simulink library "halin"  (R2021b)
settings: Solver=VariableStepAuto  StartTime=0.0  StopTime=10.0  RelTol=1e-3
undefined symbols (not defined in the file): KHAL_CAN1ABM1E2E_flg, KHAL_CAN1ESC1E2E_flg, KHAL_CAN1ESC5E2E_flg, KHAL_CAN1ESC7E2E_flg, KHAL_CAN1FCM2E2E_flg, KHAL_CAN1FCM3E2E_flg, KHAL_CAN1FCM4E2E_flg, KHAL_CAN3BMS1E2E_flg, KHAL_CAN3BMS6E2E_flg, KHAL_CAN3CCU1E2E_flg, KHAL_CAN3CCU2E2E_flg, KHAL_CAN3MCUF1E2E_flg, KHAL_CAN3MCUR1E2E_flg, KHAL_CAN3Shifter1E2E_flg, TRUE
libraries: simulink x420, FVT_lib x149, hcu_lib x49
(part 14 of 14)

== system halin/HAL_IN/CAN3/MCU_R2/RrCoolanttempReq ==
  Rr_CoolanttempReq : Inport
  UnitConverter : DataTypeConversion  OutDataTypeStr=uint16
  convert_in : FVT_lib/hal/convert_in  gain=1  offset=-40
  VHAL_RrCoolanttempReq_cnt : Outport
  wires:
  convert_in/1 -> VHAL_RrCoolanttempReq_cnt/1
  UnitConverter/1 -> convert_in/1
  Rr_CoolanttempReq/1 -> UnitConverter/1

== system halin/HAL_IN/CAN3/MCU_R2/RrEOPSpdSet ==
  Rr_EOP_SpdSet : Inport
  UnitConverter : DataTypeConversion  OutDataTypeStr=uint16
  VHAL_RrEOPSpdSet_rpm : Outport
  wires:
  UnitConverter/1 -> VHAL_RrEOPSpdSet_rpm/1
  Rr_EOP_SpdSet/1 -> UnitConverter/1

== system halin/HAL_IN/CAN3/MCU_R2/RrFailcode1 ==
  Rr_Failcode1 : Inport
  UnitConverter : DataTypeConversion  OutDataTypeStr=uint8
  VHAL_RrFailcode1_enum : Outport
  wires:
  UnitConverter/1 -> VHAL_RrFailcode1_enum/1
  Rr_Failcode1/1 -> UnitConverter/1

== system halin/HAL_IN/CAN3/MCU_R2/RrFailcode2 ==
  Rr_Failcode2 : Inport
  UnitConverter : DataTypeConversion  OutDataTypeStr=uint8
  VHAL_RrFailcode2_enum : Outport
  wires:
  UnitConverter/1 -> VHAL_RrFailcode2_enum/1
  Rr_Failcode2/1 -> UnitConverter/1

== system halin/HAL_IN/CAN3/MCU_R2/RrFailcodehistory1 ==
  Rr_Failcodehistory1 : Inport
  UnitConverter : DataTypeConversion  OutDataTypeStr=uint8
  VHAL_RrFailcodehistory1_enum : Outport
  wires:
  UnitConverter/1 -> VHAL_RrFailcodehistory1_enum/1
  Rr_Failcodehistory1/1 -> UnitConverter/1

== system halin/HAL_IN/CAN3/MCU_R2/RrFailcodehistory2 ==
  Rr_Failcodehistory2 : Inport
  UnitConverter : DataTypeConversion  OutDataTypeStr=uint8
  VHAL_RrFailcodehistory2_enum : Outport
  wires:
  UnitConverter/1 -> VHAL_RrFailcodehistory2_enum/1
  Rr_Failcodehistory2/1 -> UnitConverter/1

== system halin/HAL_IN/CAN3/MCU_R2/RrLLCTemp ==
  Rr_LLCTemp : Inport
  UnitConverter : DataTypeConversion  OutDataTypeStr=uint16
  convert_in : FVT_lib/hal/convert_in  gain=1  offset=-40
  VHAL_RrLLCTemp_C : Outport
  wires:
  convert_in/1 -> VHAL_RrLLCTemp_C/1
  UnitConverter/1 -> convert_in/1
  Rr_LLCTemp/1 -> UnitConverter/1

== system halin/HAL_IN/CAN3/MCU_R2/RrLLCflowReq ==
  Rr_LLCflowReq : Inport
  UnitConverter : DataTypeConversion  OutDataTypeStr=uint8
  convert_in : FVT_lib/hal/convert_in  gain=0.25  offset=0
  VHAL_RrLLCflowReq_Lpmin : Outport
  wires:
  convert_in/1 -> VHAL_RrLLCflowReq_Lpmin/1
  UnitConverter/1 -> convert_in/1
  Rr_LLCflowReq/1 -> UnitConverter/1

== system halin/HAL_IN/CAN3/MCU_R2/RrMCUTempWarn ==
  Rr_MCUTempWarn : Inport
  UnitConverter : DataTypeConversion  OutDataTypeStr=uint8
  VHAL_RrMCUTempWarn_enum : Outport
  wires:
  UnitConverter/1 -> VHAL_RrMCUTempWarn_enum/1
  Rr_MCUTempWarn/1 -> UnitConverter/1

== system halin/HAL_IN/CAN3/MCU_R2/RrTMTempWarn ==
  Rr_TMTempWarn : Inport
  UnitConverter : DataTypeConversion  OutDataTypeStr=uint8
  VHAL_RrTMTempWarn_enum : Outport
  wires:
  UnitConverter/1 -> VHAL_RrTMTempWarn_enum/1
  Rr_TMTempWarn/1 -> UnitConverter/1

== system halin/HAL_IN/CAN3/Shifter1/ShifterCRC8 ==
  Shifter_CRC8 : Inport
  UnitConverter : DataTypeConversion  OutDataTypeStr=uint8
  VHAL_ShifterCRC8_enum : Outport
  wires:
  UnitConverter/1 -> VHAL_ShifterCRC8_enum/1
  Shifter_CRC8/1 -> UnitConverter/1

== system halin/HAL_IN/CAN3/Shifter1/ShifterHandleCmd ==
  Shifter_Handle_Cmd : Inport
  UnitConverter : DataTypeConversion  OutDataTypeStr=uint8
  VHAL_ShifterHandleCmd_enum : Outport
  wires:
  UnitConverter/1 -> VHAL_ShifterHandleCmd_enum/1
  Shifter_Handle_Cmd/1 -> UnitConverter/1

== system halin/HAL_IN/CAN3/Shifter1/ShifterRC ==
  Shifter_RC : Inport
  UnitConverter : DataTypeConversion  OutDataTypeStr=uint8
  VHAL_ShifterRC_enum : Outport
  wires:
  UnitConverter/1 -> VHAL_ShifterRC_enum/1
  Shifter_RC/1 -> UnitConverter/1

== system halin/HAL_IN/CAN4/DKC1/DKCReVehData ==
  DKC_Re_VehData : Inport
  UnitConverter : DataTypeConversion  OutDataTypeStr=uint8
  VHAL_DKCReVehData_enum : Outport
  wires:
  UnitConverter/1 -> VHAL_DKCReVehData_enum/1
  DKC_Re_VehData/1 -> UnitConverter/1

== system halin/HAL_IN/CAN4/DKC1/DKCRemotePW ==
  DKC_Remote_PW : Inport
  UnitConverter : DataTypeConversion  OutDataTypeStr=uint8
  VHAL_DKCRemotePW_enum : Outport
  wires:
  UnitConverter/1 -> VHAL_DKCRemotePW_enum/1
  DKC_Remote_PW/1 -> UnitConverter/1

== system halin/HAL_IN/CAN4/DKC1/PCommandToBCM ==
  P_CommandToBCM : Inport
  UnitConverter : DataTypeConversion  OutDataTypeStr=uint8
  VHAL_PCommandToBCM_enum : Outport
  wires:
  UnitConverter/1 -> VHAL_PCommandToBCM_enum/1
  P_CommandToBCM/1 -> UnitConverter/1

== system halin/HAL_IN/CAN4/DKC1/PCommandToPTG ==
  P_CommandToPTG : Inport
  UnitConverter : DataTypeConversion  OutDataTypeStr=uint8
  VHAL_PCommandToPTG_enum : Outport
  wires:
  UnitConverter/1 -> VHAL_PCommandToPTG_enum/1
  P_CommandToPTG/1 -> UnitConverter/1

== system halin/HAL_IN/CAN4/DKC1/PDKeyAreaLockUnlock ==
  P_DKey_Area_LockUnlock : Inport
  UnitConverter : DataTypeConversion  OutDataTypeStr=uint8
  VHAL_PDKeyAreaLockUnlock_enum : Outport
  wires:
  UnitConverter/1 -> VHAL_PDKeyAreaLockUnlock_enum/1
  P_DKey_Area_LockUnlock/1 -> UnitConverter/1

== system halin/HAL_IN/CAN4/DKC1/PDKeyAreaPS ==
  P_DKey_Area_PS : Inport
  UnitConverter : DataTypeConversion  OutDataTypeStr=uint8
  VHAL_PDKeyAreaPS_enum : Outport
  wires:
  UnitConverter/1 -> VHAL_PDKeyAreaPS_enum/1
  P_DKey_Area_PS/1 -> UnitConverter/1

== system halin/HAL_IN/CAN4/DKC1/PDKeyAreaPTG ==
  P_DKey_Area_PTG : Inport
  UnitConverter : DataTypeConversion  OutDataTypeStr=uint8
  VHAL_PDKeyAreaPTG_enum : Outport
  wires:
  UnitConverter/1 -> VHAL_PDKeyAreaPTG_enum/1
  P_DKey_Area_PTG/1 -> UnitConverter/1

== system halin/HAL_IN/CAN4/DKC1/PDKeyWelcome ==
  P_DKey_Welcome : Inport
  UnitConverter : DataTypeConversion  OutDataTypeStr=uint8
  VHAL_PDKeyWelcome_enum : Outport
  wires:
  UnitConverter/1 -> VHAL_PDKeyWelcome_enum/1
  P_DKey_Welcome/1 -> UnitConverter/1

== system halin/HAL_IN/CAN4/DKC1/PDkeyShowIVI ==
  P_Dkey_Show_IVI : Inport
  UnitConverter : DataTypeConversion  OutDataTypeStr=uint8
  VHAL_PDkeyShowIVI_enum : Outport
  wires:
  UnitConverter/1 -> VHAL_PDkeyShowIVI_enum/1
  P_Dkey_Show_IVI/1 -> UnitConverter/1

== system halin/HAL_IN/CAN4/DKC1/PKeyMiss ==
  P_KeyMiss : Inport
  UnitConverter : DataTypeConversion  OutDataTypeStr=uint8
  VHAL_PKeyMiss_flg : Outport
  wires:
  UnitConverter/1 -> VHAL_PKeyMiss_flg/1
  P_KeyMiss/1 -> UnitConverter/1

== system halin/HAL_IN/CAN4/DKC1/PKeyMode ==
  P_KeyMode : Inport
  UnitConverter : DataTypeConversion  OutDataTypeStr=uint8
  VHAL_PKeyMode_enum : Outport
  wires:
  UnitConverter/1 -> VHAL_PKeyMode_enum/1
  P_KeyMode/1 -> UnitConverter/1

== system halin/HAL_IN/CAN4/DKC1/PUIDLowPower ==
  P_UID_LowPower : Inport
  UnitConverter : DataTypeConversion  OutDataTypeStr=uint8
  VHAL_PUIDLowPower_flg : Outport
  wires:
  UnitConverter/1 -> VHAL_PUIDLowPower_flg/1
  P_UID_LowPower/1 -> UnitConverter/1

== system halin/HAL_IN/CAN4/DKC2/EncryptionDATA063 ==
  EncryptionDATA_0_63 : Inport
  UnitConverter : DataTypeConversion  OutDataTypeStr=uint64
  VHAL_EncryptionDATA063_enum : Outport
  wires:
  UnitConverter/1 -> VHAL_EncryptionDATA063_enum/1
  EncryptionDATA_0_63/1 -> UnitConverter/1

== system halin/HAL_IN/CAN4/DKC2/EncryptionDATA64127 ==
  EncryptionDATA_64_127 : Inport
  UnitConverter : DataTypeConversion  OutDataTypeStr=uint64
  VHAL_EncryptionDATA64127_enum : Outport
  wires:
  UnitConverter/1 -> VHAL_EncryptionDATA64127_enum/1
  EncryptionDATA_64_127/1 -> UnitConverter/1

== system halin/HAL_IN/CAN4/DKC2/RandomNumberX ==
  Random_Number_X : Inport
  UnitConverter : DataTypeConversion  OutDataTypeStr=uint64
  VHAL_RandomNumberX_enum : Outport
  wires:
  UnitConverter/1 -> VHAL_RandomNumberX_enum/1
  Random_Number_X/1 -> UnitConverter/1

== system halin/HAL_IN/CAN4/GW_ZDR_PTG1/PTGRDILSta ==
  PTG_RDIL_Sta : Inport
  UnitConverter : DataTypeConversion  OutDataTypeStr=uint8
  VHAL_PTGRDILSta_enum : Outport
  wires:
  UnitConverter/1 -> VHAL_PTGRDILSta_enum/1
  PTG_RDIL_Sta/1 -> UnitConverter/1

== system halin/HAL_IN/CAN4/GW_ZoneDR1/CSWDimSw ==
  CSW_DimSw : Inport
  UnitConverter : DataTypeConversion  OutDataTypeStr=uint8
  VHAL_CSWDimSw_flg : Outport
  wires:
  UnitConverter/1 -> VHAL_CSWDimSw_flg/1
  CSW_DimSw/1 -> UnitConverter/1

== system halin/HAL_IN/CAN4/GW_ZoneDR1/CSWFWasSwSta ==
  CSW_FWasSw_Sta : Inport
  UnitConverter : DataTypeConversion  OutDataTypeStr=uint8
  VHAL_CSWFWasSwSta_enum : Outport
  wires:
  UnitConverter/1 -> VHAL_CSWFWasSwSta_enum/1
  CSW_FWasSw_Sta/1 -> UnitConverter/1

== system halin/HAL_IN/CAN4/GW_ZoneDR1/CSWFWipSwSta ==
  CSW_FWipSw_Sta : Inport
  UnitConverter : DataTypeConversion  OutDataTypeStr=uint8
  VHAL_CSWFWipSwSta_enum : Outport
  wires:
  UnitConverter/1 -> VHAL_CSWFWipSwSta_enum/1
  CSW_FWipSw_Sta/1 -> UnitConverter/1

== system halin/HAL_IN/CAN4/GW_ZoneDR1/CSWPassSWSta ==
  CSW_PassSW_Sta : Inport
  UnitConverter : DataTypeConversion  OutDataTypeStr=uint8
  VHAL_CSWPassSWSta_flg : Outport
  wires:
  UnitConverter/1 -> VHAL_CSWPassSWSta_flg/1
  CSW_PassSW_Sta/1 -> UnitConverter/1

== system halin/HAL_IN/CAN4/GW_ZoneDR1/CSWRWasSWSta ==
  CSW_RWasSW_Sta : Inport
  UnitConverter : DataTypeConversion  OutDataTypeStr=uint8
  VHAL_CSWRWasSWSta_enum : Outport
  wires:
  UnitConverter/1 -> VHAL_CSWRWasSWSta_enum/1
  CSW_RWasSW_Sta/1 -> UnitConverter/1

== system halin/HAL_IN/CAN4/GW_ZoneDR1/CSWRWipIntSwSta ==
  CSW_RWipIntSw_Sta : Inport
  UnitConverter : DataTypeConversion  OutDataTypeStr=uint8
  VHAL_CSWRWipIntSwSta_enum : Outport
  wires:
  UnitConverter/1 -> VHAL_CSWRWipIntSwSta_enum/1
  CSW_RWipIntSw_Sta/1 -> UnitConverter/1

== system halin/HAL_IN/CAN4/GW_ZoneDR1/CSWTurnSwSta ==
  CSW_TurnSw_Sta : Inport
  UnitConverter : DataTypeConversion  OutDataTypeStr=uint8
  VHAL_CSWTurnSwSta_enum : Outport
  wires:
  UnitConverter/1 -> VHAL_CSWTurnSwSta_enum/1
  CSW_TurnSw_Sta/1 -> UnitConverter/1

== system halin/HAL_IN/CAN4/GW_ZoneDR1/DrLockSta ==
  DrLockSta : Inport
  UnitConverter : DataTypeConversion  OutDataTypeStr=uint8
  VHAL_DrLockSta_flg : Outport
  wires:
  UnitConverter/1 -> VHAL_DrLockSta_flg/1
  DrLockSta/1 -> UnitConverter/1

== system halin/HAL_IN/CAN4/GW_ZoneDR1/MIRRORFOLDSW ==
  MIRROR_FOLD_SW : Inport
  UnitConverter : DataTypeConversion  OutDataTypeStr=uint8
  VHAL_MIRRORFOLDSW_flg : Outport
  wires:
  UnitConverter/1 -> VHAL_MIRRORFOLDSW_flg/1
  MIRROR_FOLD_SW/1 -> UnitConverter/1

== system halin/HAL_IN/CAN4/GW_ZoneDR1/RLSLampSta ==
  RLS_Lamp_Sta : Inport
  UnitConverter : DataTypeConversion  OutDataTypeStr=uint8
  VHAL_RLSLampSta_flg : Outport
  wires:
  UnitConverter/1 -> VHAL_RLSLampSta_flg/1
  RLS_Lamp_Sta/1 -> UnitConverter/1

== system halin/HAL_IN/CAN4/GW_ZoneDR1/RLSRainSnrWiperCmd ==
  RLS_RainSnrWiperCmd : Inport
  UnitConverter : DataTypeConversion  OutDataTypeStr=uint8
  VHAL_RLSRainSnrWiperCmd_enum : Outport
  wires:
  UnitConverter/1 -> VHAL_RLSRainSnrWiperCmd_enum/1
  RLS_RainSnrWiperCmd/1 -> UnitConverter/1

== system halin/HAL_IN/CAN4/GW_ZoneDR1/RLTurnLampC ==
  RLTurnLampC : Inport
  UnitConverter : DataTypeConversion  OutDataTypeStr=uint8
  convert_in : FVT_lib/hal/convert_in  gain=10  offset=0
  VHAL_RLTurnLampC_mA : Outport
  wires:
  convert_in/1 -> VHAL_RLTurnLampC_mA/1
  UnitConverter/1 -> convert_in/1
  RLTurnLampC/1 -> UnitConverter/1

== system halin/HAL_IN/CAN4/GW_ZoneDR1/RRTurnLampC ==
  RRTurnLampC : Inport
  UnitConverter : DataTypeConversion  OutDataTypeStr=uint8
  convert_in : FVT_lib/hal/convert_in  gain=10  offset=0
  VHAL_RRTurnLampC_mA : Outport
  wires:
  convert_in/1 -> VHAL_RRTurnLampC_mA/1
  UnitConverter/1 -> convert_in/1
  RRTurnLampC/1 -> UnitConverter/1

== system halin/HAL_IN/CAN4/GW_ZoneDR1/RWiperAS ==
  RWiperAS : Inport
  UnitConverter : DataTypeConversion  OutDataTypeStr=uint8
  VHAL_RWiperAS_flg : Outport
  wires:
  UnitConverter/1 -> VHAL_RWiperAS_flg/1
  RWiperAS/1 -> UnitConverter/1

== system halin/HAL_IN/CAN4/GW_ZoneDR1/RWiperProtection ==
  RWiperProtection : Inport
  UnitConverter : DataTypeConversion  OutDataTypeStr=uint8
  VHAL_RWiperProtection_flg : Outport
  wires:
  UnitConverter/1 -> VHAL_RWiperProtection_flg/1
  RWiperProtection/1 -> UnitConverter/1

== system halin/HAL_IN/CAN4/GW_ZoneDR2/SWCCANCELSta ==
  SWC_CANCEL_Sta : Inport
  UnitConverter : DataTypeConversion  OutDataTypeStr=uint8
  VHAL_SWCCANCELSta_flg : Outport
  wires:
  UnitConverter/1 -> VHAL_SWCCANCELSta_flg/1
  SWC_CANCEL_Sta/1 -> UnitConverter/1

== system halin/HAL_IN/CAN4/GW_ZoneDR2/SWCResUpSta ==
  SWC_Res_Up_Sta : Inport
  UnitConverter : DataTypeConversion  OutDataTypeStr=uint8
  VHAL_SWCResUpSta_flg : Outport
  wires:
  UnitConverter/1 -> VHAL_SWCResUpSta_flg/1
  SWC_Res_Up_Sta/1 -> UnitConverter/1

== system halin/HAL_IN/CAN4/GW_ZoneDR2/SWCSetdownSta ==
  SWC_Set_down_Sta : Inport
  UnitConverter : DataTypeConversion  OutDataTypeStr=uint8
  VHAL_SWCSetdownSta_flg : Outport
  wires:
  UnitConverter/1 -> VHAL_SWCSetdownSta_flg/1
  SWC_Set_down_Sta/1 -> UnitConverter/1

== system halin/HAL_IN/CAN4/GW_ZoneDR2/SWCmodeSta ==
  SWC_mode_Sta : Inport
  UnitConverter : DataTypeConversion  OutDataTypeStr=uint8
  VHAL_SWCmodeSta_flg : Outport
  wires:
  UnitConverter/1 -> VHAL_SWCmodeSta_flg/1
  SWC_mode_Sta/1 -> UnitConverter/1

== system halin/HAL_IN/CAN4/GW_ZoneDR3/LDrvValWdwOpened ==
  L_Drv_Val_Wdw_Opened : Inport
  UnitConverter : DataTypeConversion  OutDataTypeStr=uint8
  VHAL_LDrvValWdwOpened_pct : Outport
  wires:
  UnitConverter/1 -> VHAL_LDrvValWdwOpened_pct/1
  L_Drv_Val_Wdw_Opened/1 -> UnitConverter/1

== system halin/HAL_IN/CAN4/GW_ZoneDR3/LPasValWdwOpened ==
  L_Pas_Val_Wdw_Opened : Inport
  UnitConverter : DataTypeConversion  OutDataTypeStr=uint8
  VHAL_LPasValWdwOpened_pct : Outport
  wires:
  UnitConverter/1 -> VHAL_LPasValWdwOpened_pct/1
  L_Pas_Val_Wdw_Opened/1 -> UnitConverter/1

== system halin/HAL_IN/CAN4/GW_ZoneDR4/LRLDValWdwOpened ==
  L_RLD_Val_Wdw_Opened : Inport
  UnitConverter : DataTypeConversion  OutDataTypeStr=uint8
  VHAL_LRLDValWdwOpened_pct : Outport
  wires:
  UnitConverter/1 -> VHAL_LRLDValWdwOpened_pct/1
  L_RLD_Val_Wdw_Opened/1 -> UnitConverter/1

== system halin/HAL_IN/CAN4/GW_ZoneDR4/LRRDValWdwOpened ==
  L_RRD_Val_Wdw_Opened : Inport
  UnitConverter : DataTypeConversion  OutDataTypeStr=uint8
  VHAL_LRRDValWdwOpened_pct : Outport
  wires:
  UnitConverter/1 -> VHAL_LRRDValWdwOpened_pct/1
  L_RRD_Val_Wdw_Opened/1 -> UnitConverter/1

== system halin/HAL_IN/CAN4/GW_ZoneDR4/PTGInnerSW2 ==
  PTG_Inner_SW_2 : Inport
  UnitConverter : DataTypeConversion  OutDataTypeStr=uint8
  VHAL_PTGInnerSW2_enum : Outport
  wires:
  UnitConverter/1 -> VHAL_PTGInnerSW2_enum/1
  PTG_Inner_SW_2/1 -> UnitConverter/1

== system halin/HAL_IN/CAN4/GW_ZoneDR6/FrntPTCRearLeActHeatPwr ==
  FrntPTCRearLeActHeatPwr : Inport
  UnitConverter : DataTypeConversion  OutDataTypeStr=uint8
  convert_in : FVT_lib/hal/convert_in  gain=25  offset=0
  VHAL_FrntPTCRearLeActHeatPwr_W : Outport
  wires:
  convert_in/1 -> VHAL_FrntPTCRearLeActHeatPwr_W/1
  UnitConverter/1 -> convert_in/1
  FrntPTCRearLeActHeatPwr/1 -> UnitConverter/1

== system halin/HAL_IN/CAN4/GW_ZoneDR6/FrntPTCRearRiActHeatPwr ==
  FrntPTCRearRiActHeatPwr : Inport
  UnitConverter : DataTypeConversion  OutDataTypeStr=uint8
  convert_in : FVT_lib/hal/convert_in  gain=25  offset=0
  VHAL_FrntPTCRearRiActHeatPwr_W : Outport
  wires:
  convert_in/1 -> VHAL_FrntPTCRearRiActHeatPwr_W/1
  UnitConverter/1 -> convert_in/1
  FrntPTCRearRiActHeatPwr/1 -> UnitConverter/1

== system halin/HAL_IN/CAN4/GW_ZoneDR6/FrntPTCRiActHeatPwr ==
  FrntPTCRiActHeatPwr : Inport
  UnitConverter : DataTypeConversion  OutDataTypeStr=uint8
  convert_in : FVT_lib/hal/convert_in  gain=25  offset=0
  VHAL_FrntPTCRiActHeatPwr_W : Outport
  wires:
  convert_in/1 -> VHAL_FrntPTCRiActHeatPwr_W/1
  UnitConverter/1 -> convert_in/1
  FrntPTCRiActHeatPwr/1 -> UnitConverter/1

== system halin/HAL_IN/CAN4/GW_ZoneFR1/FLTurnLampC ==
  FLTurnLampC : Inport
  UnitConverter : DataTypeConversion  OutDataTypeStr=uint8
  convert_in : FVT_lib/hal/convert_in  gain=10  offset=0
  VHAL_FLTurnLampC_mA : Outport
  wires:
  convert_in/1 -> VHAL_FLTurnLampC_mA/1
  UnitConverter/1 -> convert_in/1
  FLTurnLampC/1 -> UnitConverter/1

== system halin/HAL_IN/CAN4/GW_ZoneFR1/FRTurnLampC ==
  FRTurnLampC : Inport
  UnitConverter : DataTypeConversion  OutDataTypeStr=uint8
  convert_in : FVT_lib/hal/convert_in  gain=10  offset=0
  VHAL_FRTurnLampC_mA : Outport
  wires:
  convert_in/1 -> VHAL_FRTurnLampC_mA/1
  UnitConverter/1 -> convert_in/1
  FRTurnLampC/1 -> UnitConverter/1

== system halin/HAL_IN/CAN4/GW_ZoneFR1/FWiperAS ==
  FWiperAS : Inport
  UnitConverter : DataTypeConversion  OutDataTypeStr=uint8
  VHAL_FWiperAS_flg : Outport
  wires:
  UnitConverter/1 -> VHAL_FWiperAS_flg/1
  FWiperAS/1 -> UnitConverter/1

== system halin/HAL_IN/CAN4/GW_ZoneFR1/FWiperProtection ==
  FWiperProtection : Inport
  UnitConverter : DataTypeConversion  OutDataTypeStr=uint8
  VHAL_FWiperProtection_flg : Outport
  wires:
  UnitConverter/1 -> VHAL_FWiperProtection_flg/1
  FWiperProtection/1 -> UnitConverter/1

== system halin/HAL_IN/CAN4/GW_ZoneFR2/COMPStatorSpd ==
  COMP_StatorSpd : Inport
  UnitConverter : DataTypeConversion  OutDataTypeStr=uint16
  VHAL_COMPStatorSpd_rpm : Outport
  wires:
  UnitConverter/1 -> VHAL_COMPStatorSpd_rpm/1
  COMP_StatorSpd/1 -> UnitConverter/1

== system halin/HAL_IN/CAN4/GW_ZoneFR2/CompProEN ==
  CompProEN : Inport
  UnitConverter : DataTypeConversion  OutDataTypeStr=uint8
  VHAL_CompProEN_flg : Outport
  wires:
  UnitConverter/1 -> VHAL_CompProEN_flg/1
  CompProEN/1 -> UnitConverter/1

== system halin/HAL_IN/CAN4/Zone_Dr_SCP/DrSCPSysErrLmp ==
  DrSCPSysErrLmp : Inport
  UnitConverter : DataTypeConversion  OutDataTypeStr=uint8
  VHAL_DrSCPSysErrLmp_flg : Outport
  wires:
  UnitConverter/1 -> VHAL_DrSCPSysErrLmp_flg/1
  DrSCPSysErrLmp/1 -> UnitConverter/1

== system halin/HAL_IN/CAN4/Zone_Dr_SCP/RegenMode ==
  RegenMode : Inport
  UnitConverter : DataTypeConversion  OutDataTypeStr=uint8
  VHAL_RegenMode_enum : Outport
  wires:
  UnitConverter/1 -> VHAL_RegenMode_enum/1
  RegenMode/1 -> UnitConverter/1

== system halin/HAL_IN/CAN4/Zone_Dr_SCP/SetSpd ==
  Set_Spd : Inport
  UnitConverter : DataTypeConversion  OutDataTypeStr=uint8
  VHAL_SetSpd_kph : Outport
  wires:
  UnitConverter/1 -> VHAL_SetSpd_kph/1
  Set_Spd/1 -> UnitConverter/1

== system halin/HAL_IN/CAN4/Zone_Dr_SCP/ZoneSpdCtrlMode ==
  Zone_Spd_Ctrl_Mode : Inport
  UnitConverter : DataTypeConversion  OutDataTypeStr=uint8
  VHAL_ZoneSpdCtrlMode_enum : Outport
  wires:
  UnitConverter/1 -> VHAL_ZoneSpdCtrlMode_enum/1
  Zone_Spd_Ctrl_Mode/1 -> UnitConverter/1

== system halin/HAL_IN/CAN4/Zone_Dr_THCM/BlowerErr ==
  Blower_Err : Inport
  UnitConverter : DataTypeConversion  OutDataTypeStr=uint8
  VHAL_BlowerErr_enum : Outport
  wires:
  UnitConverter/1 -> VHAL_BlowerErr_enum/1
  Blower_Err/1 -> UnitConverter/1

== system halin/HAL_IN/CAN4/Zone_Dr_THCM/SolarL ==
  SolarL : Inport
  UnitConverter : DataTypeConversion  OutDataTypeStr=uint8
  convert_in : FVT_lib/hal/convert_in  gain=5  offset=0
  VHAL_SolarL_W : Outport
  wires:
  convert_in/1 -> VHAL_SolarL_W/1
  UnitConverter/1 -> convert_in/1
  SolarL/1 -> UnitConverter/1

== system halin/HAL_IN/CAN4/Zone_Dr_THCM/SolarLErr ==
  SolarL_Err : Inport
  UnitConverter : DataTypeConversion  OutDataTypeStr=uint8
  VHAL_SolarLErr_enum : Outport
  wires:
  UnitConverter/1 -> VHAL_SolarLErr_enum/1
  SolarL_Err/1 -> UnitConverter/1

== system halin/HAL_IN/CAN4/Zone_Dr_THCM/SolarR ==
  SolarR : Inport
  UnitConverter : DataTypeConversion  OutDataTypeStr=uint8
  convert_in : FVT_lib/hal/convert_in  gain=5  offset=0
  VHAL_SolarR_W : Outport
  wires:
  convert_in/1 -> VHAL_SolarR_W/1
  UnitConverter/1 -> convert_in/1
  SolarR/1 -> UnitConverter/1

== system halin/HAL_IN/CAN4/Zone_Dr_THCM/SolarRErr ==
  SolarR_Err : Inport
  UnitConverter : DataTypeConversion  OutDataTypeStr=uint8
  VHAL_SolarRErr_enum : Outport
  wires:
  UnitConverter/1 -> VHAL_SolarRErr_enum/1
  SolarR_Err/1 -> UnitConverter/1

== system halin/HAL_IN/CAN4/Zone_Dr_THCM/TFaceL ==
  T_Face_L : Inport
  UnitConverter : DataTypeConversion  OutDataTypeStr=uint8
  convert_in : FVT_lib/hal/convert_in  gain=0.5  offset=-40
  VHAL_TFaceL_C : Outport
  wires:
  convert_in/1 -> VHAL_TFaceL_C/1
  UnitConverter/1 -> convert_in/1
  T_Face_L/1 -> UnitConverter/1

== system halin/HAL_IN/CAN4/Zone_Dr_THCM/TFaceLErr ==
  T_Face_L_Err : Inport
  UnitConverter : DataTypeConversion  OutDataTypeStr=uint8
  VHAL_TFaceLErr_enum : Outport
  wires:
  UnitConverter/1 -> VHAL_TFaceLErr_enum/1
  T_Face_L_Err/1 -> UnitConverter/1

== system halin/HAL_IN/CAN4/Zone_Dr_THCM/TFaceR ==
  T_Face_R : Inport
  UnitConverter : DataTypeConversion  OutDataTypeStr=uint8
  convert_in : FVT_lib/hal/convert_in  gain=0.5  offset=-40
  VHAL_TFaceR_C : Outport
  wires:
  convert_in/1 -> VHAL_TFaceR_C/1
  UnitConverter/1 -> convert_in/1
  T_Face_R/1 -> UnitConverter/1

== system halin/HAL_IN/CAN4/Zone_Dr_THCM/TFaceRErr ==
  T_Face_R_Err : Inport
  UnitConverter : DataTypeConversion  OutDataTypeStr=uint8
  VHAL_TFaceRErr_enum : Outport
  wires:
  UnitConverter/1 -> VHAL_TFaceRErr_enum/1
  T_Face_R_Err/1 -> UnitConverter/1

== system halin/HAL_IN/CAN4/Zone_Dr_THCM/TFaceRr ==
  T_Face_Rr : Inport
  UnitConverter : DataTypeConversion  OutDataTypeStr=uint8
  convert_in : FVT_lib/hal/convert_in  gain=0.5  offset=-40
  VHAL_TFaceRr_C : Outport
  wires:
  convert_in/1 -> VHAL_TFaceRr_C/1
  UnitConverter/1 -> convert_in/1
  T_Face_Rr/1 -> UnitConverter/1

== system halin/HAL_IN/CAN4/Zone_Dr_THCM/TFaceRrErr ==
  T_Face_Rr_Err : Inport
  UnitConverter : DataTypeConversion  OutDataTypeStr=uint8
  VHAL_TFaceRrErr_enum : Outport
  wires:
  UnitConverter/1 -> VHAL_TFaceRrErr_enum/1
  T_Face_Rr_Err/1 -> UnitConverter/1

== system halin/HAL_IN/CAN4/Zone_Dr_THCM/TFootL ==
  T_Foot_L : Inport
  UnitConverter : DataTypeConversion  OutDataTypeStr=uint8
  convert_in : FVT_lib/hal/convert_in  gain=0.5  offset=-40
  VHAL_TFootL_C : Outport
  wires:
  convert_in/1 -> VHAL_TFootL_C/1
  UnitConverter/1 -> convert_in/1
  T_Foot_L/1 -> UnitConverter/1

== system halin/HAL_IN/CAN4/Zone_Dr_THCM/TFootLErr ==
  T_Foot_L_Err : Inport
  UnitConverter : DataTypeConversion  OutDataTypeStr=uint8
  VHAL_TFootLErr_enum : Outport
  wires:
  UnitConverter/1 -> VHAL_TFootLErr_enum/1
  T_Foot_L_Err/1 -> UnitConverter/1

== system halin/HAL_IN/CAN4/Zone_Dr_THCM/TFootR ==
  T_Foot_R : Inport
  UnitConverter : DataTypeConversion  OutDataTypeStr=uint8
  convert_in : FVT_lib/hal/convert_in  gain=0.5  offset=-40
  VHAL_TFootR_C : Outport
  wires:
  convert_in/1 -> VHAL_TFootR_C/1
  UnitConverter/1 -> convert_in/1
  T_Foot_R/1 -> UnitConverter/1

== system halin/HAL_IN/CAN4/Zone_Dr_THCM/TFootRErr ==
  T_Foot_R_Err : Inport
  UnitConverter : DataTypeConversion  OutDataTypeStr=uint8
  VHAL_TFootRErr_enum : Outport
  wires:
  UnitConverter/1 -> VHAL_TFootRErr_enum/1
  T_Foot_R_Err/1 -> UnitConverter/1

== system halin/HAL_IN/CAN4/Zone_Dr_THCM/TFootRr ==
  T_Foot_Rr : Inport
  UnitConverter : DataTypeConversion  OutDataTypeStr=uint8
  convert_in : FVT_lib/hal/convert_in  gain=0.5  offset=-40
  VHAL_TFootRr_C : Outport
  wires:
  convert_in/1 -> VHAL_TFootRr_C/1
  UnitConverter/1 -> convert_in/1
  T_Foot_Rr/1 -> UnitConverter/1

== system halin/HAL_IN/CAN4/Zone_Dr_THCM/TFootRrErr ==
  T_Foot_Rr_Err : Inport
  UnitConverter : DataTypeConversion  OutDataTypeStr=uint8
  VHAL_TFootRrErr_enum : Outport
  wires:
  UnitConverter/1 -> VHAL_TFootRrErr_enum/1
  T_Foot_Rr_Err/1 -> UnitConverter/1

== system halin/HAL_IN/CAN4/Zone_Dr_THCM/Tevap ==
  Tevap : Inport
  UnitConverter : DataTypeConversion  OutDataTypeStr=uint8
  convert_in : FVT_lib/hal/convert_in  gain=0.5  offset=-40
  VHAL_Tevap_C : Outport
  wires:
  convert_in/1 -> VHAL_Tevap_C/1
  UnitConverter/1 -> convert_in/1
  Tevap/1 -> UnitConverter/1

== system halin/HAL_IN/CAN4/Zone_Dr_THCM/TevapErr ==
  Tevap_Err : Inport
  UnitConverter : DataTypeConversion  OutDataTypeStr=uint8
  VHAL_TevapErr_enum : Outport
  wires:
  UnitConverter/1 -> VHAL_TevapErr_enum/1
  Tevap_Err/1 -> UnitConverter/1

== system halin/HAL_IN/CAN4/Zone_Dr_THCM/Tincar ==
  Tincar : Inport
  UnitConverter : DataTypeConversion  OutDataTypeStr=uint8
  convert_in : FVT_lib/hal/convert_in  gain=0.5  offset=-40
  VHAL_Tincar_C : Outport
  wires:
  convert_in/1 -> VHAL_Tincar_C/1
  UnitConverter/1 -> convert_in/1
  Tincar/1 -> UnitConverter/1

== system halin/HAL_IN/CAN4/Zone_Dr_THCM/TincarErr ==
  Tincar_Err : Inport
  UnitConverter : DataTypeConversion  OutDataTypeStr=uint8
  VHAL_TincarErr_enum : Outport
  wires:
  UnitConverter/1 -> VHAL_TincarErr_enum/1
  Tincar_Err/1 -> UnitConverter/1

== system halin/HAL_IN/CAN4/Zone_Dr_VCU/DrAuBoxPwrN1Curr ==
  DrAuBoxPwrN1Curr : Inport
  UnitConverter : DataTypeConversion  OutDataTypeStr=uint8
  convert_in : FVT_lib/hal/convert_in  gain=0.125  offset=0
  VHAL_DrAuBoxPwrN1Curr_A : Outport
  wires:
  convert_in/1 -> VHAL_DrAuBoxPwrN1Curr_A/1
  UnitConverter/1 -> convert_in/1
  DrAuBoxPwrN1Curr/1 -> UnitConverter/1

== system halin/HAL_IN/CAN4/Zone_Dr_VCU/DrAuBoxPwrN2Curr ==
  DrAuBoxPwrN2Curr : Inport
  UnitConverter : DataTypeConversion  OutDataTypeStr=uint8
  convert_in : FVT_lib/hal/convert_in  gain=0.125  offset=0
  VHAL_DrAuBoxPwrN2Curr_A : Outport
  wires:
  convert_in/1 -> VHAL_DrAuBoxPwrN2Curr_A/1
  UnitConverter/1 -> convert_in/1
  DrAuBoxPwrN2Curr/1 -> UnitConverter/1

== system halin/HAL_IN/CAN4/Zone_Dr_VCU/DrColumnSWFault ==
  DrColumnSWFault : Inport
  UnitConverter : DataTypeConversion  OutDataTypeStr=uint8
  VHAL_DrColumnSWFault_enum : Outport
  wires:
  UnitConverter/1 -> VHAL_DrColumnSWFault_enum/1
  DrColumnSWFault/1 -> UnitConverter/1

== system halin/HAL_IN/CAN4/Zone_Dr_VCU/DrCtrlBDVolt ==
  DrCtrlBDVolt : Inport
  UnitConverter : DataTypeConversion  OutDataTypeStr=uint16
  convert_in : FVT_lib/hal/convert_in  gain=0.01  offset=0
  VHAL_DrCtrlBDVolt_V : Outport
  wires:
  convert_in/1 -> VHAL_DrCtrlBDVolt_V/1
  UnitConverter/1 -> convert_in/1
  DrCtrlBDVolt/1 -> UnitConverter/1

== system halin/HAL_IN/CAN4/Zone_Dr_VCU/DrCtrlTemp ==
  DrCtrlTemp : Inport
  UnitConverter : DataTypeConversion  OutDataTypeStr=uint16
  convert_in : FVT_lib/hal/convert_in  gain=0.01  offset=-40
  VHAL_DrCtrlTemp_C : Outport
  wires:
  convert_in/1 -> VHAL_DrCtrlTemp_C/1
  UnitConverter/1 -> convert_in/1
  DrCtrlTemp/1 -> UnitConverter/1

== system halin/HAL_IN/CAN4/Zone_Dr_VCU/DrEOBDFault ==
  DrEOBDFault : Inport
  UnitConverter : DataTypeConversion  OutDataTypeStr=uint8
  VHAL_DrEOBDFault_enum : Outport
  wires:
  UnitConverter/1 -> VHAL_DrEOBDFault_enum/1
  DrEOBDFault/1 -> UnitConverter/1

== system halin/HAL_IN/CAN4/Zone_Dr_VCU/DrIVIFault ==
  DrIVIFault : Inport
  UnitConverter : DataTypeConversion  OutDataTypeStr=uint8
  VHAL_DrIVIFault_enum : Outport
  wires:
  UnitConverter/1 -> VHAL_DrIVIFault_enum/1
  DrIVIFault/1 -> UnitConverter/1

== system halin/HAL_IN/CAN4/Zone_Dr_VCU/DrInfoFault ==
  DrInfoFault : Inport
  UnitConverter : DataTypeConversion  OutDataTypeStr=uint8
  VHAL_DrInfoFault_enum : Outport
  wires:
  UnitConverter/1 -> VHAL_DrInfoFault_enum/1
  DrInfoFault/1 -> UnitConverter/1

== system halin/HAL_IN/CAN4/Zone_Dr_VCU/DrPMMLVOutPErrLmp ==
  DrPMMLVOutPErrLmp : Inport
  UnitConverter : DataTypeConversion  OutDataTypeStr=uint8
  VHAL_DrPMMLVOutPErrLmp_flg : Outport
  wires:
  UnitConverter/1 -> VHAL_DrPMMLVOutPErrLmp_flg/1
  DrPMMLVOutPErrLmp/1 -> UnitConverter/1

== system halin/HAL_IN/CAN4/Zone_Dr_VCU/DrPMMLimpHomeActReq ==
  DrPMMLimpHomeActReq : Inport
  UnitConverter : DataTypeConversion  OutDataTypeStr=uint8
  VHAL_DrPMMLimpHomeActReq_flg : Outport
  wires:
  UnitConverter/1 -> VHAL_DrPMMLimpHomeActReq_flg/1
  DrPMMLimpHomeActReq/1 -> UnitConverter/1

== system halin/HAL_IN/CAN4/Zone_Dr_VCU/DrPMMSysErrLmp ==
  DrPMMSysErrLmp : Inport
  UnitConverter : DataTypeConversion  OutDataTypeStr=uint8
  VHAL_DrPMMSysErrLmp_flg : Outport
  wires:
  UnitConverter/1 -> VHAL_DrPMMSysErrLmp_flg/1
  DrPMMSysErrLmp/1 -> UnitConverter/1

== system halin/HAL_IN/CAN4/Zone_Dr_VCU/DrPowerTemp1 ==
  DrPowerTemp1 : Inport
  UnitConverter : DataTypeConversion  OutDataTypeStr=uint16
  convert_in : FVT_lib/hal/convert_in  gain=0.01  offset=-40
  VHAL_DrPowerTemp1_C : Outport
  wires:
  convert_in/1 -> VHAL_DrPowerTemp1_C/1
  UnitConverter/1 -> convert_in/1
  DrPowerTemp1/1 -> UnitConverter/1

== system halin/HAL_IN/CAN4/Zone_Dr_VCU/DrPowerTemp2 ==
  DrPowerTemp2 : Inport
  UnitConverter : DataTypeConversion  OutDataTypeStr=uint16
  convert_in : FVT_lib/hal/convert_in  gain=0.01  offset=-40
  VHAL_DrPowerTemp2_C : Outport
  wires:
  convert_in/1 -> VHAL_DrPowerTemp2_C/1
  UnitConverter/1 -> convert_in/1
  DrPowerTemp2/1 -> UnitConverter/1

== system halin/HAL_IN/CAN4/Zone_Dr_VCU/DrPwrInformationSta ==
  DrPwrInformationSta : Inport
  UnitConverter : DataTypeConversion  OutDataTypeStr=uint8
  VHAL_DrPwrInformationSta_flg : Outport
  wires:
  UnitConverter/1 -> VHAL_DrPwrInformationSta_flg/1
  DrPwrInformationSta/1 -> UnitConverter/1

== system halin/HAL_IN/CAN4/Zone_Dr_VCU/DrPwrONA1Curr ==
  DrPwrONA1Curr : Inport
  UnitConverter : DataTypeConversion  OutDataTypeStr=uint8
  convert_in : FVT_lib/hal/convert_in  gain=0.125  offset=0
  VHAL_DrPwrONA1Curr_A : Outport
  wires:
  convert_in/1 -> VHAL_DrPwrONA1Curr_A/1
  UnitConverter/1 -> convert_in/1
  DrPwrONA1Curr/1 -> UnitConverter/1

== system halin/HAL_IN/CAN4/Zone_Dr_VCU/DrPwrONA2Curr ==
  DrPwrONA2Curr : Inport
  UnitConverter : DataTypeConversion  OutDataTypeStr=uint8
  convert_in : FVT_lib/hal/convert_in  gain=0.125  offset=0
  VHAL_DrPwrONA2Curr_A : Outport
  wires:
  convert_in/1 -> VHAL_DrPwrONA2Curr_A/1
  UnitConverter/1 -> convert_in/1
  DrPwrONA2Curr/1 -> UnitConverter/1

== system halin/HAL_IN/CAN4/Zone_Dr_VCU/DrPwrSta ==
  DrPwrSta : Inport
  UnitConverter : DataTypeConversion  OutDataTypeStr=uint8
  VHAL_DrPwrSta_enum : Outport
  wires:
  UnitConverter/1 -> VHAL_DrPwrSta_enum/1
  DrPwrSta/1 -> UnitConverter/1

== system halin/HAL_IN/CAN4/Zone_Dr_VCU/DrPwrStdbyACurr ==
  DrPwrStdbyACurr : Inport
  UnitConverter : DataTypeConversion  OutDataTypeStr=uint8
  convert_in : FVT_lib/hal/convert_in  gain=0.125  offset=0
  VHAL_DrPwrStdbyACurr_A : Outport
  wires:
  convert_in/1 -> VHAL_DrPwrStdbyACurr_A/1
  UnitConverter/1 -> convert_in/1
  DrPwrStdbyACurr/1 -> UnitConverter/1

== system halin/HAL_IN/CAN4/Zone_Dr_VCU/DrPwrWindowECUFault ==
  DrPwrWindowECUFault : Inport
  UnitConverter : DataTypeConversion  OutDataTypeStr=uint8
  VHAL_DrPwrWindowECUFault_enum : Outport
  wires:
  UnitConverter/1 -> VHAL_DrPwrWindowECUFault_enum/1
  DrPwrWindowECUFault/1 -> UnitConverter/1

== system halin/HAL_IN/CAN4/Zone_Dr_VCU/DrStdAErrSta ==
  DrStdAErrSta : Inport
  UnitConverter : DataTypeConversion  OutDataTypeStr=uint8
  VHAL_DrStdAErrSta_flg : Outport
  wires:
  UnitConverter/1 -> VHAL_DrStdAErrSta_flg/1
  DrStdAErrSta/1 -> UnitConverter/1

== system halin/HAL_IN/CAN4/Zone_Dr_VCU/DrTHCMFault ==
  DrTHCMFault : Inport
  UnitConverter : DataTypeConversion  OutDataTypeStr=uint8
  VHAL_DrTHCMFault_enum : Outport
  wires:
  UnitConverter/1 -> VHAL_DrTHCMFault_enum/1
  DrTHCMFault/1 -> UnitConverter/1

== system halin/HAL_IN/CAN4/Zone_Dr_VCU/ZoneDrMalfunLevel ==
  ZoneDrMalfunLevel : Inport
  UnitConverter : DataTypeConversion  OutDataTypeStr=uint8
  VHAL_ZoneDrMalfunLevel_enum : Outport
  wires:
  UnitConverter/1 -> VHAL_ZoneDrMalfunLevel_enum/1
  ZoneDrMalfunLevel/1 -> UnitConverter/1

== system halin/HAL_IN/CAN4/Zone_Fr_THCM/AGSErr ==
  AGS_Err : Inport
  UnitConverter : DataTypeConversion  OutDataTypeStr=uint8
  VHAL_AGSErr_enum : Outport
  wires:
  UnitConverter/1 -> VHAL_AGSErr_enum/1
  AGS_Err/1 -> UnitConverter/1

== system halin/HAL_IN/CAN4/Zone_Fr_THCM/BatInTemp ==
  Bat_In_Temp : Inport
  UnitConverter : DataTypeConversion  OutDataTypeStr=uint8
  convert_in : FVT_lib/hal/convert_in  gain=0.5  offset=-40
  VHAL_BatInTemp_C : Outport
  wires:
  convert_in/1 -> VHAL_BatInTemp_C/1
  UnitConverter/1 -> convert_in/1
  Bat_In_Temp/1 -> UnitConverter/1

== system halin/HAL_IN/CAN4/Zone_Fr_THCM/BatInTempErr ==
  Bat_In_Temp_Err : Inport
  UnitConverter : DataTypeConversion  OutDataTypeStr=uint8
  VHAL_BatInTempErr_enum : Outport
  wires:
  UnitConverter/1 -> VHAL_BatInTempErr_enum/1
  Bat_In_Temp_Err/1 -> UnitConverter/1

== system halin/HAL_IN/CAN4/Zone_Fr_THCM/BatOutTemp ==
  Bat_Out_Temp : Inport
  UnitConverter : DataTypeConversion  OutDataTypeStr=uint8
  convert_in : FVT_lib/hal/convert_in  gain=0.5  offset=-40
  VHAL_BatOutTemp_C : Outport
  wires:
  convert_in/1 -> VHAL_BatOutTemp_C/1
  UnitConverter/1 -> convert_in/1
  Bat_Out_Temp/1 -> UnitConverter/1

== system halin/HAL_IN/CAN4/Zone_Fr_THCM/COMPErr ==
  COMP_Err : Inport
  UnitConverter : DataTypeConversion  OutDataTypeStr=uint8
  VHAL_COMPErr_enum : Outport
  wires:
  UnitConverter/1 -> VHAL_COMPErr_enum/1
  COMP_Err/1 -> UnitConverter/1

== system halin/HAL_IN/CAN4/Zone_Fr_THCM/EACProtectEnable ==
  EACProtectEnable : Inport
  UnitConverter : DataTypeConversion  OutDataTypeStr=uint8
  VHAL_EACProtectEnable_enum : Outport
  wires:
  UnitConverter/1 -> VHAL_EACProtectEnable_enum/1
  EACProtectEnable/1 -> UnitConverter/1

== system halin/HAL_IN/CAN4/Zone_Fr_THCM/EWP3Err ==
  EWP3_Err : Inport
  UnitConverter : DataTypeConversion  OutDataTypeStr=uint8
  VHAL_EWP3Err_enum : Outport
  wires:
  UnitConverter/1 -> VHAL_EWP3Err_enum/1
  EWP3_Err/1 -> UnitConverter/1

== system halin/HAL_IN/CAN4/Zone_Fr_THCM/EXV1Err ==
  EXV1_Err : Inport
  UnitConverter : DataTypeConversion  OutDataTypeStr=uint8
  VHAL_EXV1Err_enum : Outport
  wires:
  UnitConverter/1 -> VHAL_EXV1Err_enum/1
  EXV1_Err/1 -> UnitConverter/1

== system halin/HAL_IN/CAN4/Zone_Fr_THCM/EXV2Err ==
  EXV2_Err : Inport
  UnitConverter : DataTypeConversion  OutDataTypeStr=uint8
  VHAL_EXV2Err_enum : Outport
  wires:
  UnitConverter/1 -> VHAL_EXV2Err_enum/1
  EXV2_Err/1 -> UnitConverter/1

== system halin/HAL_IN/CAN4/Zone_Fr_THCM/FanErr ==
  Fan_Err : Inport
  UnitConverter : DataTypeConversion  OutDataTypeStr=uint8
  VHAL_FanErr_enum : Outport
  wires:
  UnitConverter/1 -> VHAL_FanErr_enum/1
  Fan_Err/1 -> UnitConverter/1

== system halin/HAL_IN/CAN4/Zone_Fr_THCM/MotorInTemp ==
  Motor_In_Temp : Inport
  UnitConverter : DataTypeConversion  OutDataTypeStr=uint8
  convert_in : FVT_lib/hal/convert_in  gain=0.5  offset=-40
  VHAL_MotorInTemp_C : Outport
  wires:
  convert_in/1 -> VHAL_MotorInTemp_C/1
  UnitConverter/1 -> convert_in/1
  Motor_In_Temp/1 -> UnitConverter/1

== system halin/HAL_IN/CAN4/Zone_Fr_THCM/MotorInTempErr ==
  Motor_In_Temp_Err : Inport
  UnitConverter : DataTypeConversion  OutDataTypeStr=uint8
  VHAL_MotorInTempErr_enum : Outport
  wires:
  UnitConverter/1 -> VHAL_MotorInTempErr_enum/1
  Motor_In_Temp_Err/1 -> UnitConverter/1

== system halin/HAL_IN/CAN4/Zone_Fr_THCM/MotorOutTemp ==
  Motor_Out_Temp : Inport
  UnitConverter : DataTypeConversion  OutDataTypeStr=uint8
  convert_in : FVT_lib/hal/convert_in  gain=0.5  offset=-40
  VHAL_MotorOutTemp_C : Outport
  wires:
  convert_in/1 -> VHAL_MotorOutTemp_C/1
  UnitConverter/1 -> convert_in/1
  Motor_Out_Temp/1 -> UnitConverter/1

== system halin/HAL_IN/CAN4/Zone_Fr_THCM/MotorOutTempErr ==
  Motor_Out_Temp_Err : Inport
  UnitConverter : DataTypeConversion  OutDataTypeStr=uint8
  VHAL_MotorOutTempErr_enum : Outport
  wires:
  UnitConverter/1 -> VHAL_MotorOutTempErr_enum/1
  Motor_Out_Temp_Err/1 -> UnitConverter/1

== system halin/HAL_IN/CAN4/Zone_Fr_THCM/PTHighP ==
  PT_High_P : Inport
  UnitConverter : DataTypeConversion  OutDataTypeStr=uint16
  VHAL_PTHighP_KPa : Outport
  wires:
  UnitConverter/1 -> VHAL_PTHighP_KPa/1
  PT_High_P/1 -> UnitConverter/1

== system halin/HAL_IN/CAN4/Zone_Fr_THCM/PTHighPErr ==
  PT_High_P_Err : Inport
  UnitConverter : DataTypeConversion  OutDataTypeStr=uint8
  VHAL_PTHighPErr_enum : Outport
  wires:
  UnitConverter/1 -> VHAL_PTHighPErr_enum/1
  PT_High_P_Err/1 -> UnitConverter/1

== system halin/HAL_IN/CAN4/Zone_Fr_THCM/PTHighTact ==
  PT_High_Tact : Inport
  UnitConverter : DataTypeConversion  OutDataTypeStr=uint8
  convert_in : FVT_lib/hal/convert_in  gain=1  offset=-40
  VHAL_PTHighTact_C : Outport
  wires:
  convert_in/1 -> VHAL_PTHighTact_C/1
  UnitConverter/1 -> convert_in/1
  PT_High_Tact/1 -> UnitConverter/1

== system halin/HAL_IN/CAN4/Zone_Fr_THCM/PTHighTactErr ==
  PT_High_Tact_Err : Inport
  UnitConverter : DataTypeConversion  OutDataTypeStr=uint8
  VHAL_PTHighTactErr_enum : Outport
  wires:
  UnitConverter/1 -> VHAL_PTHighTactErr_enum/1
  PT_High_Tact_Err/1 -> UnitConverter/1

== system halin/HAL_IN/CAN4/Zone_Fr_THCM/PTLowP1 ==
  PT_Low_P1 : Inport
  UnitConverter : DataTypeConversion  OutDataTypeStr=uint16
  VHAL_PTLowP1_KPa : Outport
  wires:
  UnitConverter/1 -> VHAL_PTLowP1_KPa/1
  PT_Low_P1/1 -> UnitConverter/1

== system halin/HAL_IN/CAN4/Zone_Fr_THCM/PTLowP1Err ==
  PT_Low_P1_Err : Inport
  UnitConverter : DataTypeConversion  OutDataTypeStr=uint8
  VHAL_PTLowP1Err_enum : Outport
  wires:
  UnitConverter/1 -> VHAL_PTLowP1Err_enum/1
  PT_Low_P1_Err/1 -> UnitConverter/1

== system halin/HAL_IN/CAN4/Zone_Fr_THCM/PTLowP2 ==
  PT_Low_P2 : Inport
  UnitConverter : DataTypeConversion  OutDataTypeStr=uint16
  VHAL_PTLowP2_KPa : Outport
  wires:
  UnitConverter/1 -> VHAL_PTLowP2_KPa/1
  PT_Low_P2/1 -> UnitConverter/1

== system halin/HAL_IN/CAN4/Zone_Fr_THCM/PTLowP2Err ==
  PT_Low_P2_Err : Inport
  UnitConverter : DataTypeConversion  OutDataTypeStr=uint8
  VHAL_PTLowP2Err_enum : Outport
  wires:
  UnitConverter/1 -> VHAL_PTLowP2Err_enum/1
  PT_Low_P2_Err/1 -> UnitConverter/1

== system halin/HAL_IN/CAN4/Zone_Fr_THCM/PTLowT1 ==
  PT_Low_T1 : Inport
  UnitConverter : DataTypeConversion  OutDataTypeStr=uint8
  convert_in : FVT_lib/hal/convert_in  gain=0.5  offset=-40
  VHAL_PTLowT1_C : Outport
  wires:
  convert_in/1 -> VHAL_PTLowT1_C/1
  UnitConverter/1 -> convert_in/1
  PT_Low_T1/1 -> UnitConverter/1

== system halin/HAL_IN/CAN4/Zone_Fr_THCM/PTLowT1Err ==
  PT_Low_T1_Err : Inport
  UnitConverter : DataTypeConversion  OutDataTypeStr=uint8
  VHAL_PTLowT1Err_enum : Outport
  wires:
  UnitConverter/1 -> VHAL_PTLowT1Err_enum/1
  PT_Low_T1_Err/1 -> UnitConverter/1

== system halin/HAL_IN/CAN4/Zone_Fr_THCM/PTLowT2 ==
  PT_Low_T2 : Inport
  UnitConverter : DataTypeConversion  OutDataTypeStr=uint8
  convert_in : FVT_lib/hal/convert_in  gain=0.5  offset=-40
  VHAL_PTLowT2_C : Outport
  wires:
  convert_in/1 -> VHAL_PTLowT2_C/1
  UnitConverter/1 -> convert_in/1
  PT_Low_T2/1 -> UnitConverter/1

== system halin/HAL_IN/CAN4/Zone_Fr_THCM/PTLowT2Err ==
  PT_Low_T2_Err : Inport
  UnitConverter : DataTypeConversion  OutDataTypeStr=uint8
  VHAL_PTLowT2Err_enum : Outport
  wires:
  UnitConverter/1 -> VHAL_PTLowT2Err_enum/1
  PT_Low_T2_Err/1 -> UnitConverter/1

== system halin/HAL_IN/CAN4/Zone_Fr_THCM/SOTXVErr ==
  SOTXV_Err : Inport
  UnitConverter : DataTypeConversion  OutDataTypeStr=uint8
  VHAL_SOTXVErr_enum : Outport
  wires:
  UnitConverter/1 -> VHAL_SOTXVErr_enum/1
  SOTXV_Err/1 -> UnitConverter/1

== system halin/HAL_IN/CAN4/Zone_Fr_THCM/SOV1Err ==
  SOV1_Err : Inport
  UnitConverter : DataTypeConversion  OutDataTypeStr=uint8
  VHAL_SOV1Err_enum : Outport
  wires:
  UnitConverter/1 -> VHAL_SOV1Err_enum/1
  SOV1_Err/1 -> UnitConverter/1

== system halin/HAL_IN/CAN4/Zone_Fr_THCM/SOV2Err ==
  SOV2_Err : Inport
  UnitConverter : DataTypeConversion  OutDataTypeStr=uint8
  VHAL_SOV2Err_enum : Outport
  wires:
  UnitConverter/1 -> VHAL_SOV2Err_enum/1
  SOV2_Err/1 -> UnitConverter/1

== system halin/HAL_IN/CAN4/Zone_Fr_THCM/SOV3Err ==
  SOV3_Err : Inport
  UnitConverter : DataTypeConversion  OutDataTypeStr=uint8
  VHAL_SOV3Err_enum : Outport
  wires:
  UnitConverter/1 -> VHAL_SOV3Err_enum/1
  SOV3_Err/1 -> UnitConverter/1

== system halin/HAL_IN/CAN4/Zone_Fr_THCM/Tamb ==
  Tamb : Inport
  UnitConverter : DataTypeConversion  OutDataTypeStr=uint8
  convert_in : FVT_lib/hal/convert_in  gain=0.5  offset=-40
  VHAL_Tamb_C : Outport
  wires:
  convert_in/1 -> VHAL_Tamb_C/1
  UnitConverter/1 -> convert_in/1
  Tamb/1 -> UnitConverter/1

== system halin/HAL_IN/CAN4/Zone_Fr_THCM/TambErr ==
  Tamb_Err : Inport
  UnitConverter : DataTypeConversion  OutDataTypeStr=uint8
  VHAL_TambErr_enum : Outport
  wires:
  UnitConverter/1 -> VHAL_TambErr_enum/1
  Tamb_Err/1 -> UnitConverter/1

== system halin/HAL_IN/CAN5/TBOX1/PowerOffTSet ==
  PowerOff_T_Set : Inport
  UnitConverter : DataTypeConversion  OutDataTypeStr=uint8
  convert_in : FVT_lib/hal/convert_in  gain=1  offset=1
  VHAL_PowerOffTSet_cnt : Outport
  wires:
  convert_in/1 -> VHAL_PowerOffTSet_cnt/1
  UnitConverter/1 -> convert_in/1
  PowerOff_T_Set/1 -> UnitConverter/1

== system halin/HAL_IN/CAN5/TBOX1/ReDoorLock ==
  Re_DoorLock : Inport
  UnitConverter : DataTypeConversion  OutDataTypeStr=uint16
  VHAL_ReDoorLock_enum : Outport
  wires:
  UnitConverter/1 -> VHAL_ReDoorLock_enum/1
  Re_DoorLock/1 -> UnitConverter/1

== system halin/HAL_IN/CAN5/TBOX1/ReOutsideMirror ==
  ReOutsideMirror : Inport
  UnitConverter : DataTypeConversion  OutDataTypeStr=uint8
  VHAL_ReOutsideMirror_enum : Outport
  wires:
  UnitConverter/1 -> VHAL_ReOutsideMirror_enum/1
  ReOutsideMirror/1 -> UnitConverter/1

== system halin/HAL_IN/CAN5/TBOX1/RePwrReqTbox ==
  Re_PwrReqTbox : Inport
  UnitConverter : DataTypeConversion  OutDataTypeStr=uint8
  VHAL_RePwrReqTbox_enum : Outport
  wires:
  UnitConverter/1 -> VHAL_RePwrReqTbox_enum/1
  Re_PwrReqTbox/1 -> UnitConverter/1

== system halin/HAL_IN/CAN5/TBOX1/RemoteACTemp ==
  Remote_ACTemp : Inport
  UnitConverter : DataTypeConversion  OutDataTypeStr=uint8
  convert_in : FVT_lib/hal/convert_in  gain=0.5  offset=17
  VHAL_RemoteACTemp_C : Outport
  wires:
  convert_in/1 -> VHAL_RemoteACTemp_C/1
  UnitConverter/1 -> convert_in/1
  Remote_ACTemp/1 -> UnitConverter/1

== system halin/HAL_IN/CAN5/TBOX1/RemoteAutoReq ==
  Remote_AutoReq : Inport
  UnitConverter : DataTypeConversion  OutDataTypeStr=uint8
  VHAL_RemoteAutoReq_flg : Outport
  wires:
  UnitConverter/1 -> VHAL_RemoteAutoReq_flg/1
  Remote_AutoReq/1 -> UnitConverter/1
